simulink model "AUT580_twincat_communication_blocks"  (R2023a)
settings: Solver=FixedStepAuto  StartTime=0.0  StopTime=inf  FixedStep=0.002  RelTol=1e-3
settings Model: Creator=localadmin  LastModifiedBy=mustalah
settings OptimizationCC: DefaultParameterBehavior=Inlined  LocalBlockOutputs=off
settings ModelReferenceCC: EnableRefExpFcnMdlSchedulingChecks=on
settings RTWCC: Description=TwinCAT GRT Target  SystemTargetFile=TwinCatGrt.tlc  TemplateMakefile=tcgrt_msbuild.tmf  TargetLang=C++
settings STFCustomTargetCC: TargetLangStandard=C++11 (ISO)  CombineOutputUpdateFcns=on  CodeInterfacePackaging=Reusable function  CPPClassGenCompliant=on  GRTInterface=off  GenerateAllocFcn=on  UseToolchainInfoCompliant=off  SystemTargetFile=TwinCatGrt.tlc
settings GRTTargetCC: TargetLangStandard=C++11 (ISO)  ParMdlRefBuildCompliant=off  CompOptLevelCompliant=off  MatFileLogging=off  CodeInterfacePackaging=Reusable function  GenerateAllocFcn=on  UseToolchainInfoCompliant=off  ExtModeMexFile=TcExtModeClient

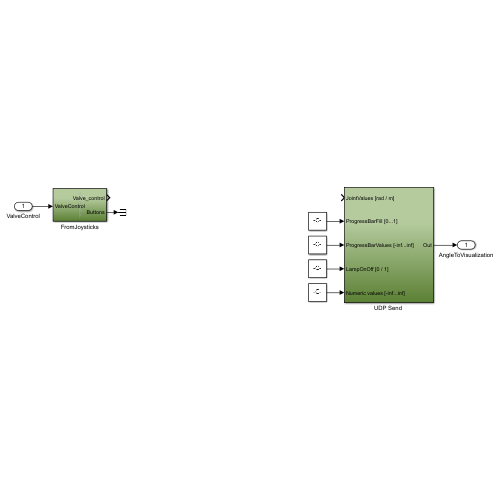
[thumbnail: Simulink's stored preview of the top-level diagram]
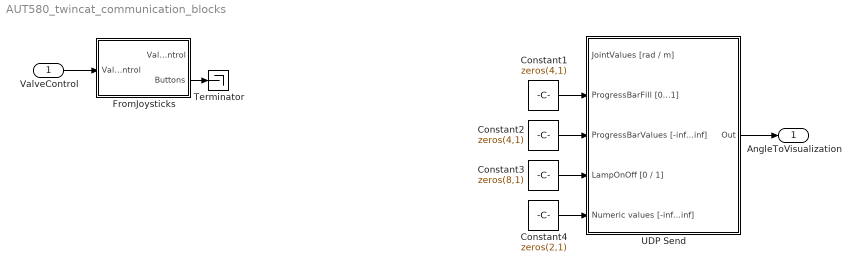
== system AUT580_twincat_communication_blocks ==
  ValveControl : Inport  OutDataTypeStr=double  PortDimensions=19
  Constant1 : Constant  Value=zeros(4,1)
  Constant2 : Constant  Value=zeros(4,1)
  Constant3 : Constant  Value=zeros(8,1)
  Constant4 : Constant  Value=zeros(2,1)
  FromJoysticks : Subsystem
  Terminator : Terminator
  "UDP Send " : Subsystem
  AngleToVisualization : Outport  OutDataTypeStr=single  PortDimensions=22
  wires:
  ValveControl/1 -> FromJoysticks/1(ValveControl)
  "UDP Send "/1(Out) -> AngleToVisualization/1
  Constant2/1 -> "UDP Send "/3(ProgressBarValues [-inf...inf])
  FromJoysticks/2(Buttons) -> Terminator/1
  Constant1/1 -> "UDP Send "/2(ProgressBarFill [0...1])
  Constant3/1 -> "UDP Send "/4(LampOnOff [0 / 1])
  Constant4/1 -> "UDP Send "/5(Numeric values [-inf...inf])

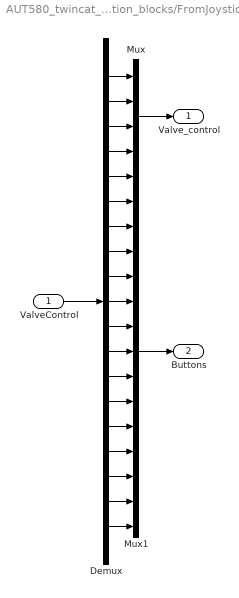
== system AUT580_twincat_communication_blocks/FromJoysticks ==
  ValveControl : Inport  OutDataTypeStr=double  PortDimensions=19
  Demux : Demux  Outputs=19
  Mux : Mux
  Mux1 : Mux  Inputs=15
  Valve_control : Outport
  Buttons : Outport  Port=2
  wires:
  ValveControl/1 -> Demux/1
  Demux/13 -> Mux1/9
  Demux/15 -> Mux1/11
  Demux/12 -> Mux1/8
  Demux/3 -> Mux/3
  Demux/11 -> Mux1/7
  Demux/16 -> Mux1/12
  Demux/14 -> Mux1/10
  Mux/1 -> Valve_control/1
  Demux/1 -> Mux/1
  Demux/9 -> Mux1/5
  Mux1/1 -> Buttons/1
  Demux/4 -> Mux/4
  Demux/6 -> Mux1/2
  Demux/2 -> Mux/2
  Demux/7 -> Mux1/3
  Demux/10 -> Mux1/6
  Demux/5 -> Mux1/1
  Demux/8 -> Mux1/4
  Demux/17 -> Mux1/13
  Demux/18 -> Mux1/14
  Demux/19 -> Mux1/15

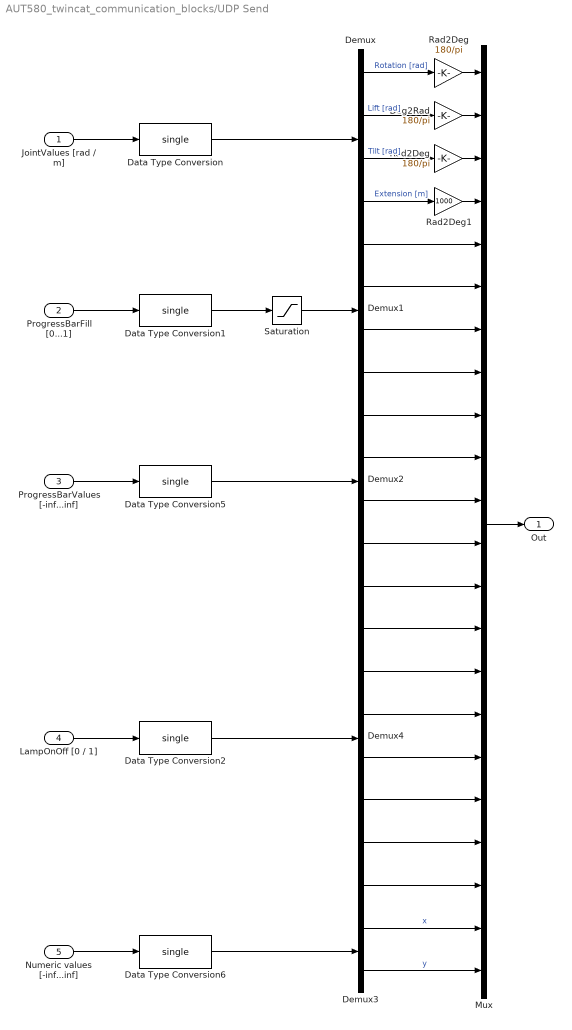
== system AUT580_twincat_communication_blocks/UDP Send  ==
  JointValues [rad / m] : Inport
  ProgressBarFill [0...1] : Inport  Port=2
  ProgressBarValues [-inf...inf] : Inport  Port=3
  LampOnOff [0 / 1] : Inport  Port=4
  Numeric values [-inf...inf] : Inport  Port=5
  Data Type Conversion{,1..2,5..6} (5 alike) : DataTypeConversion  OutDataTypeStr=single  SaturateOnIntegerOverflow=off  RndMeth=Floor
  "Deg2Rad " : Gain  Gain=180/pi
  Demux : Demux
  Demux1 : Demux
  Demux2 : Demux
  Demux3 : Demux  Outputs=2
  Demux4 : Demux  Outputs=8
  Mux : Mux  Inputs=22
  Rad2Deg : Gain  Gain=180/pi
  "Rad2Deg " : Gain  Gain=180/pi
  Rad2Deg1 : Gain  Gain=1000
  Saturation : Saturate  UpperLimit=1  LowerLimit=0
  Out : Outport  OutDataTypeStr=single  PortDimensions=22
  wires:
  JointValues [rad / m]/1 -> Data Type Conversion/1
  Demux/4 -> Rad2Deg1/1  "Extension [m]"
  Demux/2 -> "Deg2Rad "/1  "Lift [rad]"
  Demux/3 -> Rad2Deg/1  "Tilt [rad]"
  Demux/1 -> "Rad2Deg "/1  "Rotation [rad]"
  "Rad2Deg "/1 -> Mux/1
  "Deg2Rad "/1 -> Mux/2
  Rad2Deg/1 -> Mux/3
  Data Type Conversion/1 -> Demux/1
  Demux1/1 -> Mux/5
  Demux1/2 -> Mux/6
  Demux1/3 -> Mux/7
  Demux1/4 -> Mux/8
  Demux2/1 -> Mux/9
  Demux2/2 -> Mux/10
  Demux2/3 -> Mux/11
  Demux2/4 -> Mux/12
  Data Type Conversion1/1 -> Saturation/1
  Data Type Conversion5/1 -> Demux2/1
  Demux4/1 -> Mux/13
  Demux4/2 -> Mux/14
  Demux4/3 -> Mux/15
  Demux4/4 -> Mux/16
  Demux4/5 -> Mux/17
  Demux4/6 -> Mux/18
  Demux4/7 -> Mux/19
  Demux4/8 -> Mux/20
  Demux3/1 -> Mux/21  "x"
  Demux3/2 -> Mux/22  "y"
  LampOnOff [0 / 1]/1 -> Data Type Conversion2/1
  Data Type Conversion2/1 -> Demux4/1
  Saturation/1 -> Demux1/1
  ProgressBarFill [0...1]/1 -> Data Type Conversion1/1
  ProgressBarValues [-inf...inf]/1 -> Data Type Conversion5/1
  Numeric values [-inf...inf]/1 -> Data Type Conversion6/1
  Data Type Conversion6/1 -> Demux3/1
  Mux/1 -> Out/1
  Rad2Deg1/1 -> Mux/4
